simulink model "Simulink_6"  (R2013b)
settings: Solver=FixedStepDiscrete  StartTime=0.0  StopTime=1000.0  FixedStep=1  RelTol=1e-3
undefined symbols (not defined in the file or in its folder): j, magnitude
libraries: simulink x1
settings Model: ExtModeAutoUpdateStatusClock=off  Creator=asteele  LastModifiedBy=99900361
settings DataIOCC: SignalLoggingSaveFormat=ModelDataLogs  SignalLoggingName=sigsOut
settings OptimizationCC: BooleanDataType=off
settings DebuggingCC: SaveWithParameterizedLinksMsg=none  SignalResolutionControl=TryResolveAllWithWarning  SolverPrmCheckMsg=none  MultiTaskDSMMsg=warning  MultiTaskCondExecSysMsg=none  StrictBusMsg=None
settings HardwareCC: TargetUnknown=on
settings RTWCC: IncludeERTFirstTime=on
settings GRTTargetCC: CombineOutputUpdateFcns=off  GRTInterface=on

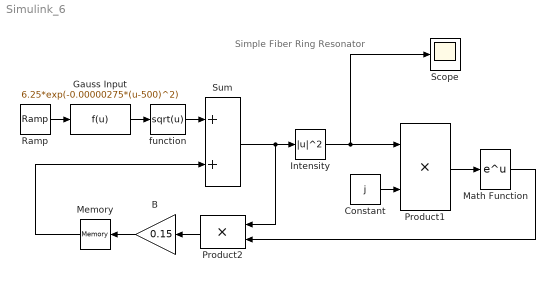
== system Simulink_6 ==
  note: Simple Fiber Ring Resonator
  B : Gain  Gain=0.15  SaturateOnIntegerOverflow=on  OutDataTypeStr=Inherit: Same as input  ParamDataTypeStr=Inherit: Same as input
  Constant : Constant  Value=j
  Gauss Input : Fcn  Expr=6.25*exp(-0.00000275*(u-500)^2)
  Intensity : Math  Operator=magnitude^2  SaturateOnIntegerOverflow=on
  Math Function : Math  SaturateOnIntegerOverflow=on
  Memory : Memory
  Product1 : Product  SaturateOnIntegerOverflow=on  InputSameDT=on  OutDataTypeStr=Inherit: Same as first input
  Product2 : Product  SaturateOnIntegerOverflow=on  InputSameDT=on  OutDataTypeStr=Inherit: Same as first input
  Ramp : simulink/Sources/Ramp  slope=1  start=0  X0=0
  Scope : Scope
  Sum : Sum  SaturateOnIntegerOverflow=on  InputSameDT=on  OutDataTypeStr=Inherit: Same as first input
  function : Fcn  Expr=sqrt(u)
  wires:
  Sum/1 -> Intensity/1, Product2/1
  Intensity/1 -> Product1/1, Scope/1
  Product2/1 -> B/1
  B/1 -> Memory/1
  Math Function/1 -> Product2/2
  Constant/1 -> Product1/2
  Product1/1 -> Math Function/1
  Memory/1 -> Sum/2
  Ramp/1 -> Gauss Input/1
  Gauss Input/1 -> function/1
  function/1 -> Sum/1
